simulink model "untitled"  (R2019b)
settings: Solver=FixedStepAuto  StartTime=0.0  StopTime=1000  FixedStep=1/1000  RelTol=1e-3
libraries: dspstat3 x10, simulink x4, simulink_extras x1
settings Model: Creator=bayra  LastModifiedBy=bayra

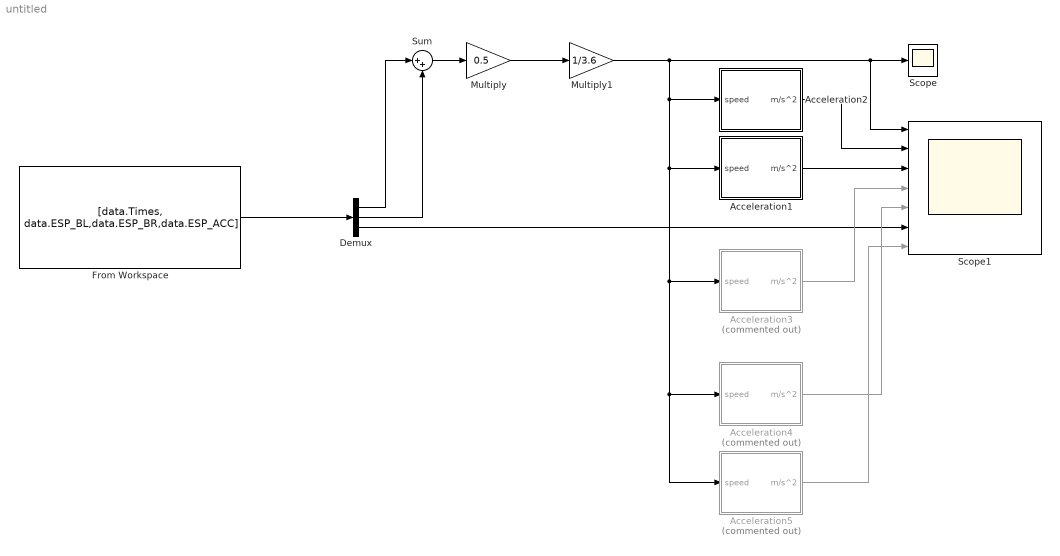
== system untitled ==
  Acceleration1 : Subsystem
  Acceleration2 : Subsystem
  Acceleration3 : Subsystem  Commented=on
  Acceleration4 : Subsystem  Commented=on
  Acceleration5 : Subsystem  Commented=on
  Demux : Demux  Outputs=3
  From Workspace : FromWorkspace  VariableName=[data.Times, data.ESP_BL,data.ESP_BR,data.ESP_ACC]
  Multiply : Gain  Gain=0.5
  Multiply1 : Gain  Gain=1/3.6
  Scope : Scope
  Scope1 : Scope  NumInputPorts=7
  Sum : Sum  Inputs=|++
  wires:
  Multiply/1 -> Multiply1/1
  Sum/1 -> Multiply/1
  From Workspace/1 -> Demux/1
  Demux/1 -> Sum/1
  Demux/2 -> Sum/2
  Acceleration1/1(m/s^2) -> Scope1/3
  Multiply1/1 -> Acceleration2/1(speed), Acceleration3/1(speed), Acceleration4/1(speed), Acceleration5/1(speed), Acceleration1/1(speed), Scope1/1, Scope/1
  Acceleration2/1(m/s^2) -> Scope1/2
  Demux/3 -> Scope1/6
  Acceleration3/1(m/s^2) -> Scope1/4
  Acceleration4/1(m/s^2) -> Scope1/5
  Acceleration5/1(m/s^2) -> Scope1/7

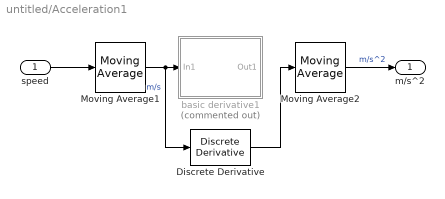
== system untitled/Acceleration1 ==
  speed : Inport
  Discrete Derivative : simulink/Discrete/Discrete Derivative  gainval=1.0  ICPrevScaledInput=0.0  OutMin=[]  OutMax=[]  OutDataType=fixdt(1, 16)  OutScaling=2^-10  DoSatur=off
  Moving Average1 : dspstat3/Moving Average  Method=Sliding window  ForgettingFactorPort=off  SpecifyWindowLength=on  WindowLength=100  ForgettingFactor=0.9  SimulateUsing=Code generation
  Moving Average2 : dspstat3/Moving Average  Method=Sliding window  ForgettingFactorPort=off  SpecifyWindowLength=on  WindowLength=100  ForgettingFactor=0.9  SimulateUsing=Code generation
  basic derivative1 : Subsystem  Commented=on
  m/s^2 : Outport
  wires:
  Moving Average2/1 -> m/s^2/1  "m/s^2"
  speed/1 -> Moving Average1/1
  Moving Average1/1 -> Discrete Derivative/1, basic derivative1/1(In1)  "m/s"
  Discrete Derivative/1 -> Moving Average2/1

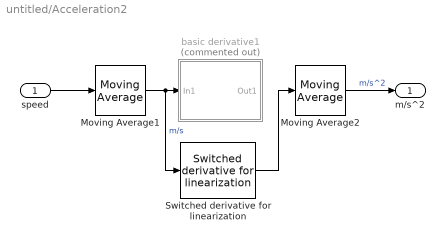
== system untitled/Acceleration2 ==
  speed : Inport
  Moving Average1 : dspstat3/Moving Average  Method=Sliding window  ForgettingFactorPort=off  SpecifyWindowLength=on  WindowLength=100  ForgettingFactor=0.9  SimulateUsing=Code generation
  Moving Average2 : dspstat3/Moving Average  Method=Sliding window  ForgettingFactorPort=off  SpecifyWindowLength=on  WindowLength=100  ForgettingFactor=0.9  SimulateUsing=Code generation
  Switched derivative for linearization : simulink_extras/Linearization/Switched derivative for linearization  switchVal=1  derivConst=10
      settings: SourceProductName=Simulink  SourceProductBaseCode=SL
  basic derivative1 : Subsystem  Commented=on
  m/s^2 : Outport
  wires:
  Switched derivative for linearization/1 -> Moving Average2/1
  Moving Average1/1 -> Switched derivative for linearization/1, basic derivative1/1(In1)  "m/s"
  speed/1 -> Moving Average1/1
  Moving Average2/1 -> m/s^2/1  "m/s^2"

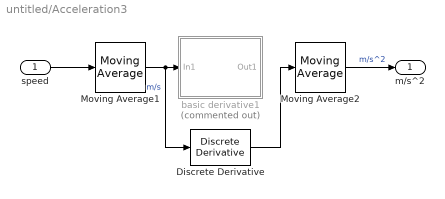
== system untitled/Acceleration3 ==
  speed : Inport
  Discrete Derivative : simulink/Discrete/Discrete Derivative  gainval=1.0  ICPrevScaledInput=0.0  OutMin=[]  OutMax=[]  OutDataType=fixdt(1, 16)  OutScaling=2^-10  DoSatur=off
  Moving Average1 : dspstat3/Moving Average  Method=Sliding window  ForgettingFactorPort=off  SpecifyWindowLength=on  WindowLength=150  ForgettingFactor=0.9  SimulateUsing=Code generation
  Moving Average2 : dspstat3/Moving Average  Method=Sliding window  ForgettingFactorPort=off  SpecifyWindowLength=on  WindowLength=150  ForgettingFactor=0.9  SimulateUsing=Code generation
  basic derivative1 : Subsystem  Commented=on
  m/s^2 : Outport
  wires:
  Discrete Derivative/1 -> Moving Average2/1
  Moving Average1/1 -> basic derivative1/1(In1), Discrete Derivative/1  "m/s"
  speed/1 -> Moving Average1/1
  Moving Average2/1 -> m/s^2/1  "m/s^2"

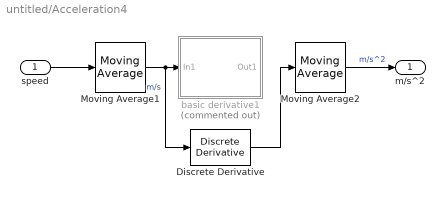
== system untitled/Acceleration4 ==
  speed : Inport
  Discrete Derivative : simulink/Discrete/Discrete Derivative  gainval=1.0  ICPrevScaledInput=0.0  OutMin=[]  OutMax=[]  OutDataType=fixdt(1, 16)  OutScaling=2^-10  DoSatur=off
  Moving Average1 : dspstat3/Moving Average  Method=Sliding window  ForgettingFactorPort=off  SpecifyWindowLength=on  WindowLength=200  ForgettingFactor=0.9  SimulateUsing=Code generation
  Moving Average2 : dspstat3/Moving Average  Method=Sliding window  ForgettingFactorPort=off  SpecifyWindowLength=on  WindowLength=200  ForgettingFactor=0.9  SimulateUsing=Code generation
  basic derivative1 : Subsystem  Commented=on
  m/s^2 : Outport
  wires:
  Moving Average2/1 -> m/s^2/1  "m/s^2"
  speed/1 -> Moving Average1/1
  Moving Average1/1 -> Discrete Derivative/1, basic derivative1/1(In1)  "m/s"
  Discrete Derivative/1 -> Moving Average2/1

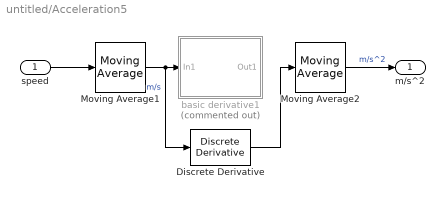
== system untitled/Acceleration5 ==
  speed : Inport
  Discrete Derivative : simulink/Discrete/Discrete Derivative  gainval=1.0  ICPrevScaledInput=0.0  OutMin=[]  OutMax=[]  OutDataType=fixdt(1, 16)  OutScaling=2^-10  DoSatur=off
  Moving Average1 : dspstat3/Moving Average  Method=Sliding window  ForgettingFactorPort=off  SpecifyWindowLength=on  WindowLength=250  ForgettingFactor=0.9  SimulateUsing=Code generation
  Moving Average2 : dspstat3/Moving Average  Method=Sliding window  ForgettingFactorPort=off  SpecifyWindowLength=on  WindowLength=250  ForgettingFactor=0.9  SimulateUsing=Code generation
  basic derivative1 : Subsystem  Commented=on
  m/s^2 : Outport
  wires:
  Discrete Derivative/1 -> Moving Average2/1
  Moving Average1/1 -> basic derivative1/1(In1), Discrete Derivative/1  "m/s"
  speed/1 -> Moving Average1/1
  Moving Average2/1 -> m/s^2/1  "m/s^2"

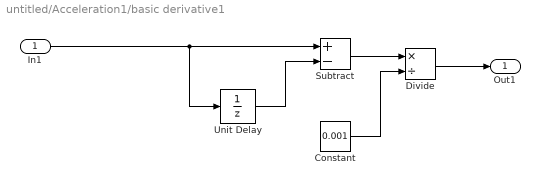
== system untitled/Acceleration1/basic derivative1 ==
  In1 : Inport
  Constant : Constant  Value=0.001  OutDataTypeStr=single
  Divide : Product  Inputs=*/
  Subtract : Sum  Inputs=+-
  Unit Delay : UnitDelay  SampleTime=-1  HasFrameUpgradeWarning=on
  Out1 : Outport
  wires:
  Unit Delay/1 -> Subtract/2
  Subtract/1 -> Divide/1
  Constant/1 -> Divide/2
  Divide/1 -> Out1/1
  In1/1 -> Subtract/1, Unit Delay/1

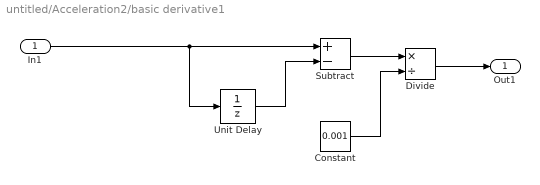
== system untitled/Acceleration2/basic derivative1 ==
  In1 : Inport
  Constant : Constant  Value=0.001  OutDataTypeStr=single
  Divide : Product  Inputs=*/
  Subtract : Sum  Inputs=+-
  Unit Delay : UnitDelay  SampleTime=-1  HasFrameUpgradeWarning=on
  Out1 : Outport
  wires:
  In1/1 -> Unit Delay/1, Subtract/1
  Divide/1 -> Out1/1
  Constant/1 -> Divide/2
  Subtract/1 -> Divide/1
  Unit Delay/1 -> Subtract/2

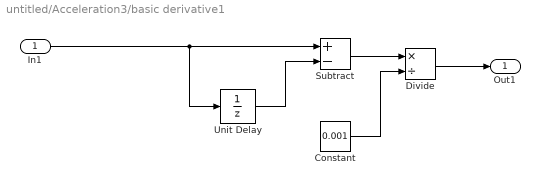
== system untitled/Acceleration3/basic derivative1 ==
  In1 : Inport
  Constant : Constant  Value=0.001  OutDataTypeStr=single
  Divide : Product  Inputs=*/
  Subtract : Sum  Inputs=+-
  Unit Delay : UnitDelay  SampleTime=-1  HasFrameUpgradeWarning=on
  Out1 : Outport
  wires:
  In1/1 -> Unit Delay/1, Subtract/1
  Divide/1 -> Out1/1
  Constant/1 -> Divide/2
  Subtract/1 -> Divide/1
  Unit Delay/1 -> Subtract/2

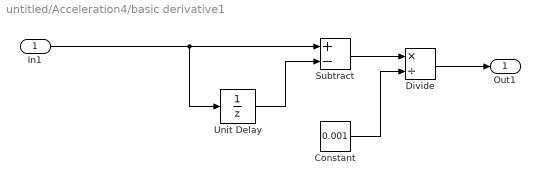
== system untitled/Acceleration4/basic derivative1 ==
  In1 : Inport
  Constant : Constant  Value=0.001  OutDataTypeStr=single
  Divide : Product  Inputs=*/
  Subtract : Sum  Inputs=+-
  Unit Delay : UnitDelay  SampleTime=-1  HasFrameUpgradeWarning=on
  Out1 : Outport
  wires:
  Unit Delay/1 -> Subtract/2
  Subtract/1 -> Divide/1
  Constant/1 -> Divide/2
  Divide/1 -> Out1/1
  In1/1 -> Subtract/1, Unit Delay/1

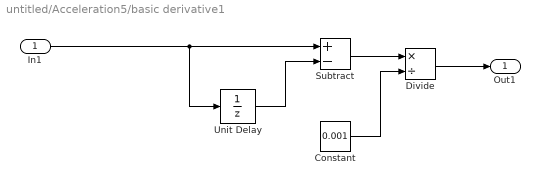
== system untitled/Acceleration5/basic derivative1 ==
  In1 : Inport
  Constant : Constant  Value=0.001  OutDataTypeStr=single
  Divide : Product  Inputs=*/
  Subtract : Sum  Inputs=+-
  Unit Delay : UnitDelay  SampleTime=-1  HasFrameUpgradeWarning=on
  Out1 : Outport
  wires:
  In1/1 -> Unit Delay/1, Subtract/1
  Divide/1 -> Out1/1
  Constant/1 -> Divide/2
  Subtract/1 -> Divide/1
  Unit Delay/1 -> Subtract/2
